simulink model "suspended_motion_test"  (R2014b)
settings: Solver=FixedStepDiscrete  StartTime=0.0  StopTime=inf  FixedStep=sample_time  RelTol=1e-3
undefined symbols (not defined in the file): A_angle_lat, A_lpf_accel, A_lpf_dtau, angle_midpoint_lat, B1_lpf_accel, B1_lpf_dtau, B2_lpf_accel, B2_lpf_dtau, back_left_triangle_period, back_left_triangle_wave_midpoint, back_left_triangle_wave_speed, back_right_triangle_period, back_right_triangle_wave_midpoint, back_right_triangle_wave_speed, boom_mount_angle, control_start_time, front_left_triangle_period, front_left_triangle_wave_midpoint, front_left_triangle_wave_speed, front_right_triangle_period, front_right_triangle_wave_midpoint, front_right_triangle_wave_speed, g, j_segments, k_ff, k_sea, kd_lateral, kd_motor, kd_sea_torque_flight, kd_sea_torque_stance, kp_lateral, kp_motor, kp_sea_torque_flight, kp_sea_torque_stance, lateral_offset, lateral_torque_ramp_time, m_leg_motor, max_sagittal_loaded_torque, max_sagittal_unloaded_torque, max_torque_lateral, maximum_lateral_angle, minimum_lateral_angle, sagittal_torque_ramp_time, sample_time, sea_control_torque_cmd_small_threshold, sea_offset_friction, sea_static_friction, stance_flight_torque_threshold, w_angle_lat
libraries: simulink x8
settings Model: xpc_rtwmakecfg_data=_xpcethercatlib_  BufferReuse=off  Creator=wmartin  LastModifiedBy=wmartin
settings SolverCC: EnableConcurrentExecution=on
settings DataIOCC: MaxDataPoints=1000000000  SaveFormat=StructureWithTime
settings OptimizationCC: BlockReduction=off  OptimizeBlockIOStorage=off  BufferReuse=off  GlobalBufferReuse=off  ExpressionFolding=off  ExpressionDepthLimit=2147483647  LocalBlockOutputs=off  SimCompilerOptimization=On
settings DebuggingCC: UnderspecifiedInitializationDetection=Classic  MergeDetectMultiDrivingBlocksExec=none  StateNameClashWarn=warning
settings HardwareCC: ProdIntDivRoundTo=Zero  ProdEndianess=LittleEndian  ProdLongLongMode=on  ProdHWDeviceType=Generic->32-bit x86 compatible
settings ModelReferenceCC: UpdateModelReferenceTargets=IfOutOfDate  EnableParallelModelReferenceBuilds=on
settings RTWCC: SystemTargetFile=slrt.tlc  TemplateMakefile=slrt_default_tmf  Description=Simulink Real-Time  RTWVerbose=off  ProcessScript=slrt_make_rtw_hook  RTWCompilerOptimization=On
settings CodeAppCC: MaxIdLength=256
settings SimulinkRealTimeCC: GeneratePreprocessorConditionals=Disable all  EnableShiftOperators=on  RL32LogBufSizeModifier=100000000

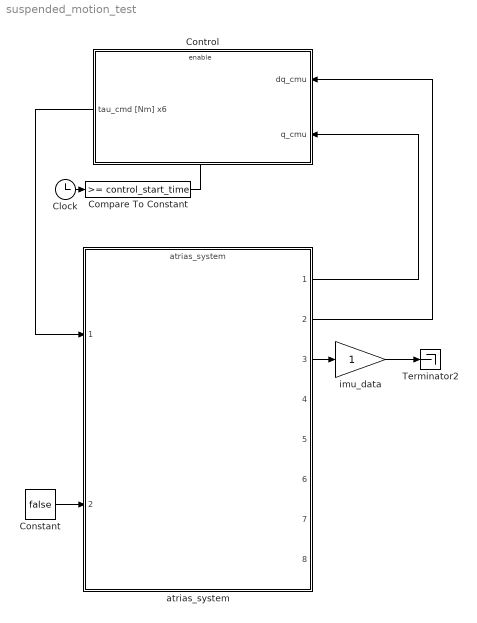
== system suspended_motion_test ==
  Clock : Clock
  Compare To Constant : simulink/Logic and Bit Operations/Compare To Constant  relop=>=  const=control_start_time  OutDataTypeStr=boolean
  Constant : Constant  Value=false
  Control : Subsystem
  Terminator2 : Terminator
  atrias_system : ModelReference  ModelNameDialog=atrias_system  SimulationMode=Normal  ModelReferenceVersion=1.2635  CopyOfModelName=atrias_system  DefaultDataLogging=on
  imu_data : Gain
  wires:
  Clock/1 -> Compare To Constant/1
  Compare To Constant/1 -> Control/Enable
  atrias_system/1 -> Control/2(q_cmu)
  atrias_system/2 -> Control/1(dq_cmu)
  Constant/1 -> atrias_system/2
  Control/1(tau_cmd [Nm] x6) -> atrias_system/1
  imu_data/1 -> Terminator2/1
  atrias_system/3 -> imu_data/1

== system suspended_motion_test/Control ==
  dq_cmu : Inport
  q_cmu : Inport  Port=2
  Enable : EnablePort  StatesWhenEnabling=reset
  Actuator Control : ModelReference  ModelNameDialog=actuator_control  SimulationMode=Normal  ModelReferenceVersion=1.25  CopyOfModelName=actuator_control  DefaultDataLogging=on
  Actuator Control old : Subsystem  Commented=on
  Behavior Control : Subsystem
  Constant : Constant  Value=[false false false false]  OutDataTypeStr=boolean
  tau_cmd [Nm] x6 : Outport  InitialOutput=[0 0 0 0 0 0]
  wires:
  q_cmu/1 -> Actuator Control/3, Behavior Control/2(q_cmu)
  dq_cmu/1 -> Actuator Control/4, Behavior Control/1(dq_cmu)
  Behavior Control/1(motor_torque_cmd) -> Actuator Control/1
  Actuator Control/1 -> tau_cmd [Nm] x6/1
  Constant/1 -> Actuator Control/2

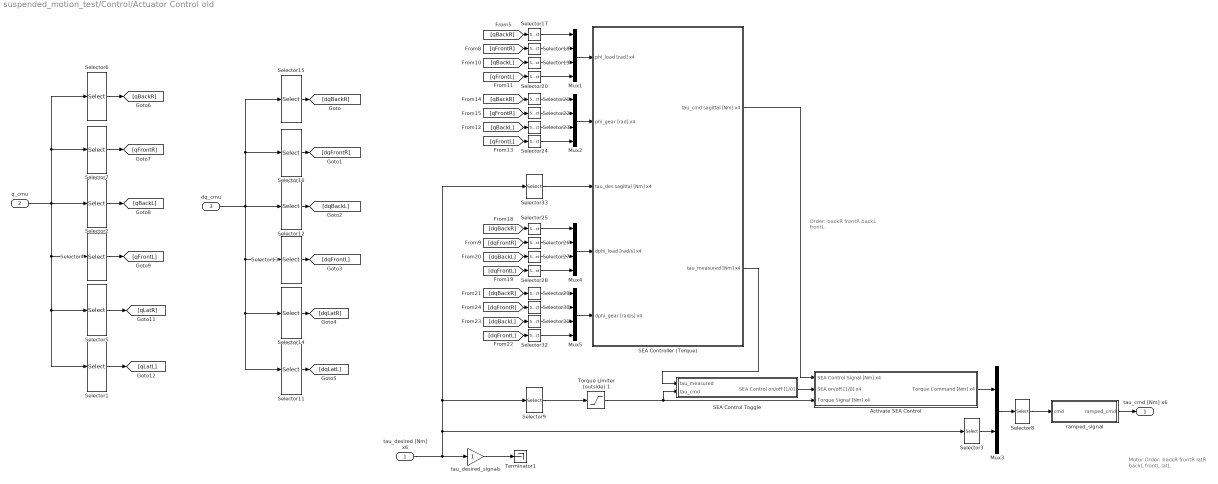
== system suspended_motion_test/Control/Actuator Control old ==
  note: Motor Order:
      |
      | backR
      | frontR
      | latR
      | backL
      | frontL
      | latL
  note: Order:
      | backR
      | frontR
      | backL
      | frontL
  tau_desired [Nm] x6 : Inport
  q_cmu : Inport  Port=2
  dq_cmu : Inport  Port=3
  Activate SEA Control : Subsystem
  Mux{1..2,4..5} (4 alike) : Mux
  Mux3 : Mux  Inputs=2
  SEA Control Toggle : Subsystem
  SEA Controller (Torque) : Subsystem
  Selector1 : Selector  InputPortWidth=13  Indices=[10]
  Selector11 : Selector  InputPortWidth=13  Indices=[10]
  Selector12 : Selector  InputPortWidth=13  Indices=[5 6]
  Selector13 : Selector  InputPortWidth=13  Indices=[7 8]
  Selector14 : Selector  InputPortWidth=13  Indices=[9]
  Selector15 : Selector  InputPortWidth=13  Indices=[1 2]
  Selector16 : Selector  InputPortWidth=13  Indices=[3 4]
  Selector{17..20,25..28} (8 alike) : Selector  InputPortWidth=2  Indices=[1]
  Selector2 : Selector  InputPortWidth=13  Indices=[5 6]
  Selector{21..24,29..32} (8 alike) : Selector  InputPortWidth=2  Indices=[2]
  Selector3 : Selector  InputPortWidth=6  Indices=[3 6]
  Selector33 : Selector  InputPortWidth=6  Indices=[1 2 4 5]
  Selector4 : Selector  InputPortWidth=13  Indices=[7 8]
  Selector5 : Selector  InputPortWidth=13  Indices=[9]
  Selector6 : Selector  InputPortWidth=13  Indices=[1 2]
  Selector7 : Selector  InputPortWidth=13  Indices=[3 4]
  Selector8 : Selector  InputPortWidth=6  Indices=[1 2 5 3 4 6]
  Selector9 : Selector  InputPortWidth=6  Indices=[1 2 4 5]
  Terminator1 : Terminator
  Torque Limiter (outside) 1 : Saturate  UpperLimit=max_sagittal_unloaded_torque  LowerLimit=-max_sagittal_unloaded_torque
      settings: AttributesFormatString=Hi: %<UpperLimit>\nLo: %<LowerLimit>
  ramped_signal : Subsystem
  tau_desired_signals : Gain  Description=xPCTag(1)=tau_cmd_signal;
  tau_cmd [Nm] x6 : Outport  InitialOutput=[0 0 0 0 0 0]
  wires:
  Mux3/1 -> Selector8/1
  Selector3/1 -> Mux3/2
  Selector33/1 -> SEA Controller (Torque)/3(tau_des sagittal [Nm] x4)
  [dqFrontL] -> Selector32/1
  [dqBackL] -> Selector31/1
  [dqFrontR] -> Selector30/1
  Selector32/1 -> Mux5/4
  Selector30/1 -> Mux5/2
  Selector31/1 -> Mux5/3
  Selector29/1 -> Mux5/1
  [dqBackR] -> Selector29/1
  Mux5/1 -> SEA Controller (Torque)/5(dphi_gear [rad/s] x4)
  [dqFrontL] -> Selector28/1
  [dqBackL] -> Selector27/1
  [dqFrontR] -> Selector26/1
  Selector28/1 -> Mux4/4
  Selector26/1 -> Mux4/2
  Selector27/1 -> Mux4/3
  Selector25/1 -> Mux4/1
  [dqBackR] -> Selector25/1
  Mux4/1 -> SEA Controller (Torque)/4(dphi_load [rad/s] x4)
  [qFrontL] -> Selector24/1
  [qBackL] -> Selector23/1
  [qFrontR] -> Selector22/1
  Selector24/1 -> Mux2/4
  Selector22/1 -> Mux2/2
  Selector23/1 -> Mux2/3
  Selector21/1 -> Mux2/1
  [qBackR] -> Selector21/1
  Mux2/1 -> SEA Controller (Torque)/2(phi_gear [rad] x4)
  [qFrontL] -> Selector20/1
  [qBackL] -> Selector19/1
  [qFrontR] -> Selector18/1
  Selector20/1 -> Mux1/4
  Selector18/1 -> Mux1/2
  Selector19/1 -> Mux1/3
  Selector17/1 -> Mux1/1
  [qBackR] -> Selector17/1
  Mux1/1 -> SEA Controller (Torque)/1(phi_load [rad] x4)
  Selector13/1 -> [dqFrontL]
  Selector12/1 -> [dqBackL]
  Selector16/1 -> [dqFrontR]
  Selector15/1 -> [dqBackR]
  Selector11/1 -> [dqLatL]
  Selector14/1 -> [dqLatR]
  dq_cmu/1 -> Selector11/1, Selector14/1, Selector13/1, Selector15/1, Selector16/1, Selector12/1
  Selector8/1 -> ramped_signal/1(cmd)
  q_cmu/1 -> Selector2/1, Selector7/1, Selector6/1, Selector4/1, Selector5/1, Selector1/1
  Selector4/1 -> [qFrontL]
  Selector2/1 -> [qBackL]
  Selector7/1 -> [qFrontR]
  Selector6/1 -> [qBackR]
  Selector1/1 -> [qLatL]
  Selector5/1 -> [qLatR]
  tau_desired_signals/1 -> Terminator1/1
  ramped_signal/1(ramped_cmd) -> tau_cmd [Nm] x6/1
  tau_desired [Nm] x6/1 -> Selector33/1, Selector9/1, Selector3/1, tau_desired_signals/1
  Activate SEA Control/1(Torque Command [Nm] x4) -> Mux3/1
  Torque Limiter (outside) 1/1 -> Activate SEA Control/3(Torque Signal [Nm] x4), SEA Control Toggle/2(tau_cmd)
  SEA Controller (Torque)/1(tau_cmd sagittal [Nm] x4) -> Activate SEA Control/1(SEA Control Signal [Nm] x4)
  SEA Control Toggle/1(SEA Control on/off [1/0]) -> Activate SEA Control/2("SEA on/off [1/0] x4 ")
  SEA Controller (Torque)/2(tau_measured [Nm] x4) -> SEA Control Toggle/1(tau_measured)
  Selector9/1 -> Torque Limiter (outside) 1/1

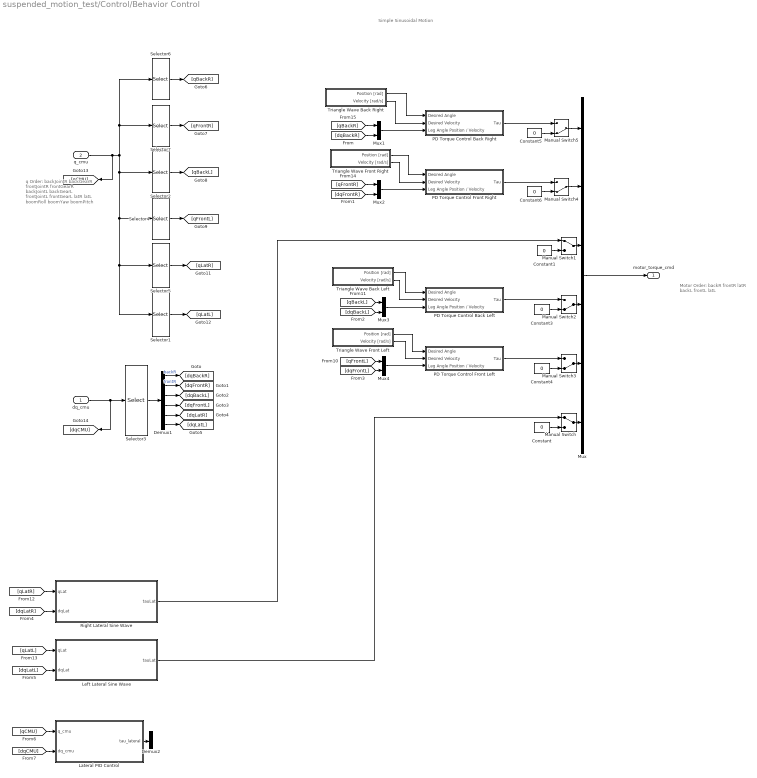
== system suspended_motion_test/Control/Behavior Control ==
  note: q Order:
      |
      | backJointR
      | backGearR
      | frontJointR
      | frontGearR
      |
      | backJointL
      | backGearL
      | frontJointL
      | frontGearL
      |
      | latR
      | latL
      |
      | boomRoll
      | boomYaw
      | boomPitch
  note: Motor Order:
      |
      | backR
      | frontR
      | latR
      | backL
      | frontL
      | latL
  note: Simple Sinusoidal Motion
  dq_cmu : Inport
  q_cmu : Inport  Port=2
  Constant{,1,3..6} (6 alike) : Constant  Value=0
  Demux1 : Demux  Outputs=6
  Demux2 : Demux  Outputs=2
  Lateral PID Control : Subsystem
  Left Lateral Sine Wave : Subsystem
  Manual Switch : ManualSwitch
  Manual Switch1 : ManualSwitch
  Manual Switch{2..5} (4 alike) : ManualSwitch  CurrentSetting=0
  Mux : Mux  Inputs=6
  Mux{1..4} (4 alike) : Mux  Inputs=2
  PD Torque Control Back Left : Subsystem
  PD Torque Control Back Right : Subsystem
  PD Torque Control Front Left : Subsystem
  PD Torque Control Front Right : Subsystem
  Right Lateral Sine Wave : Subsystem
  Selector1 : Selector  InputPortWidth=13  Indices=[10]
  Selector2 : Selector  InputPortWidth=13  Indices=[6]
  Selector3 : Selector  InputPortWidth=13  Indices=[2 4 6 8 9 10]
  Selector4 : Selector  InputPortWidth=13  Indices=[8]
  Selector5 : Selector  InputPortWidth=13  Indices=[9]
  Selector6 : Selector  InputPortWidth=13  Indices=[2]
  Selector7 : Selector  InputPortWidth=13  Indices=[4]
  Triangle Wave Back Left : Subsystem
  Triangle Wave Back Right : Subsystem
  Triangle Wave Front Left : Subsystem
  Triangle Wave Front Right : Subsystem
  motor_torque_cmd : Outport  OutputWhenDisabled=reset  InitialOutput=[0 0 0 0 0 0]
  wires:
  Mux/1 -> motor_torque_cmd/1
  dq_cmu/1 -> [dqCMU], Selector3/1
  Selector3/1 -> Demux1/1
  Left Lateral Sine Wave/1(tauLat) -> Manual Switch/1
  Manual Switch1/1 -> Mux/3
  Manual Switch/1 -> Mux/6
  Constant/1 -> Manual Switch/2
  Constant1/1 -> Manual Switch1/2
  Selector5/1 -> [qLatR]
  Selector1/1 -> [qLatL]
  Demux1/1 -> [dqBackR]  "backR"
  Demux1/2 -> [dqFrontR]  "frontR"
  Demux1/3 -> [dqBackL]
  Demux1/4 -> [dqFrontL]
  Demux1/5 -> [dqLatR]
  Demux1/6 -> [dqLatL]
  [dqLatL] -> Left Lateral Sine Wave/2(dqLat)
  Selector6/1 -> [qBackR]
  Selector7/1 -> [qFrontR]
  Selector2/1 -> [qBackL]
  Selector4/1 -> [qFrontL]
  q_cmu/1 -> [qCMU], Selector1/1, Selector5/1, Selector4/1, Selector2/1, Selector7/1, Selector6/1
  [qLatL] -> Left Lateral Sine Wave/1(qLat)
  PD Torque Control Back Right/1(Tau) -> Manual Switch5/1
  PD Torque Control Front Right/1(Tau) -> Manual Switch4/1
  Constant3/1 -> Manual Switch2/2
  Constant4/1 -> Manual Switch3/2
  Manual Switch3/1 -> Mux/5
  Manual Switch2/1 -> Mux/4
  [qBackR] -> Mux1/1
  [dqBackR] -> Mux1/2
  Mux1/1 -> PD Torque Control Back Right/3(Leg Angle Position / Velocity)
  [qFrontR] -> Mux2/1
  [dqFrontR] -> Mux2/2
  Mux2/1 -> PD Torque Control Front Right/3(Leg Angle Position / Velocity)
  [qBackL] -> Mux3/1
  [dqBackL] -> Mux3/2
  [qFrontL] -> Mux4/1
  [dqFrontL] -> Mux4/2
  Triangle Wave Front Right/1(Position [rad]) -> PD Torque Control Front Right/1(Desired Angle)
  Triangle Wave Front Right/2(Velocity [rad/s]) -> PD Torque Control Front Right/2(Desired Velocity)
  Triangle Wave Back Right/1(Position [rad]) -> PD Torque Control Back Right/1(Desired Angle)
  Triangle Wave Back Right/2(Velocity [rad/s]) -> PD Torque Control Back Right/2(Desired Velocity)
  PD Torque Control Back Left/1(Tau) -> Manual Switch2/1
  Triangle Wave Back Left/1(Position [rad]) -> PD Torque Control Back Left/1(Desired Angle)
  Triangle Wave Back Left/2(Velocity [rad/s]) -> PD Torque Control Back Left/2(Desired Velocity)
  Mux3/1 -> PD Torque Control Back Left/3(Leg Angle Position / Velocity)
  PD Torque Control Front Left/1(Tau) -> Manual Switch3/1
  Mux4/1 -> PD Torque Control Front Left/3(Leg Angle Position / Velocity)
  Triangle Wave Front Left/2(Velocity [rad/s]) -> PD Torque Control Front Left/2(Desired Velocity)
  Triangle Wave Front Left/1(Position [rad]) -> PD Torque Control Front Left/1(Desired Angle)
  Manual Switch4/1 -> Mux/2
  Manual Switch5/1 -> Mux/1
  Constant5/1 -> Manual Switch5/2
  Constant6/1 -> Manual Switch4/2
  [qLatR] -> Right Lateral Sine Wave/1(qLat)
  [dqLatR] -> Right Lateral Sine Wave/2(dqLat)
  Lateral PID Control/1(tau_lateral) -> Demux2/1
  [dqCMU] -> Lateral PID Control/2(dq_cmu)
  [qCMU] -> Lateral PID Control/1(q_cmu)
  Right Lateral Sine Wave/1(tauLat) -> Manual Switch1/1

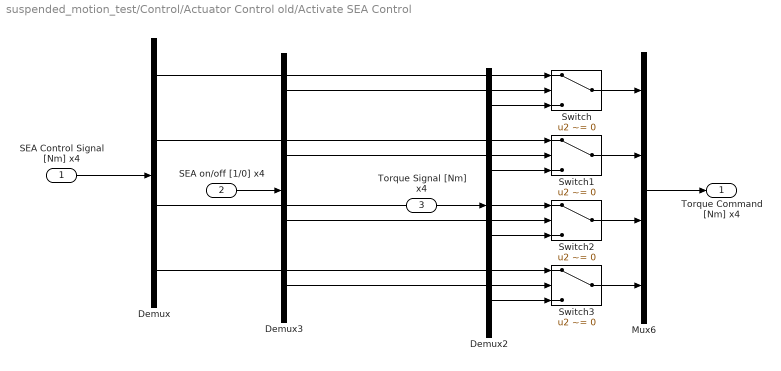
== system suspended_motion_test/Control/Actuator Control old/Activate SEA Control ==
  SEA Control Signal [Nm] x4 : Inport
  "SEA on/off [1/0] x4 " : Inport  Port=2
  Torque Signal [Nm] x4 : Inport  Port=3
  Demux : Demux
  Demux2 : Demux
  Demux3 : Demux
  Mux6 : Mux
  Switch{,1..3} (4 alike) : Switch  Criteria=u2 ~= 0
  Torque Command [Nm] x4 : Outport
  wires:
  Demux2/2 -> Switch1/3
  Demux2/1 -> Switch/3
  Demux/1 -> Switch/1
  Switch/1 -> Mux6/1
  Switch1/1 -> Mux6/2
  Switch3/1 -> Mux6/4
  Demux3/1 -> Switch/2
  Mux6/1 -> Torque Command [Nm] x4/1
  Demux3/3 -> Switch2/2
  Demux3/2 -> Switch1/2
  Demux/3 -> Switch2/1
  Switch2/1 -> Mux6/3
  Demux/4 -> Switch3/1
  Demux2/4 -> Switch3/3
  Demux3/4 -> Switch3/2
  Demux/2 -> Switch1/1
  Demux2/3 -> Switch2/3
  SEA Control Signal [Nm] x4/1 -> Demux/1
  "SEA on/off [1/0] x4 "/1 -> Demux3/1
  Torque Signal [Nm] x4/1 -> Demux2/1

== system suspended_motion_test/Control/Actuator Control old/SEA Control Toggle ==
  tau_measured : Inport
  tau_cmd : Inport  Port=2
  Abs : Abs
  Abs1 : Abs
  But Commanding a Small Torque? : simulink/Logic and Bit Operations/Compare To Constant  relop=<  const=sea_control_torque_cmd_small_threshold  OutDataTypeStr=boolean
  Logical Operator1 : Logic  AllPortsSameDT=off  OutDataTypeStr=boolean
  Logical Operator2 : Logic  Operator=NOT  AllPortsSameDT=off  OutDataTypeStr=boolean
  Measuring a Large Torque? (High Gains) : simulink/Logic and Bit Operations/Compare To Constant  relop=>=  const=stance_flight_torque_threshold  OutDataTypeStr=boolean
  SEA Control on/off [1/0] : Outport
  wires:
  Logical Operator2/1 -> SEA Control on/off [1/0]/1
  But Commanding a Small Torque?/1 -> Logical Operator1/2
  Logical Operator1/1 -> Logical Operator2/1
  tau_cmd/1 -> Abs/1
  Abs/1 -> But Commanding a Small Torque?/1
  tau_measured/1 -> Abs1/1
  Measuring a Large Torque? (High Gains)/1 -> Logical Operator1/1
  Abs1/1 -> Measuring a Large Torque? (High Gains)/1

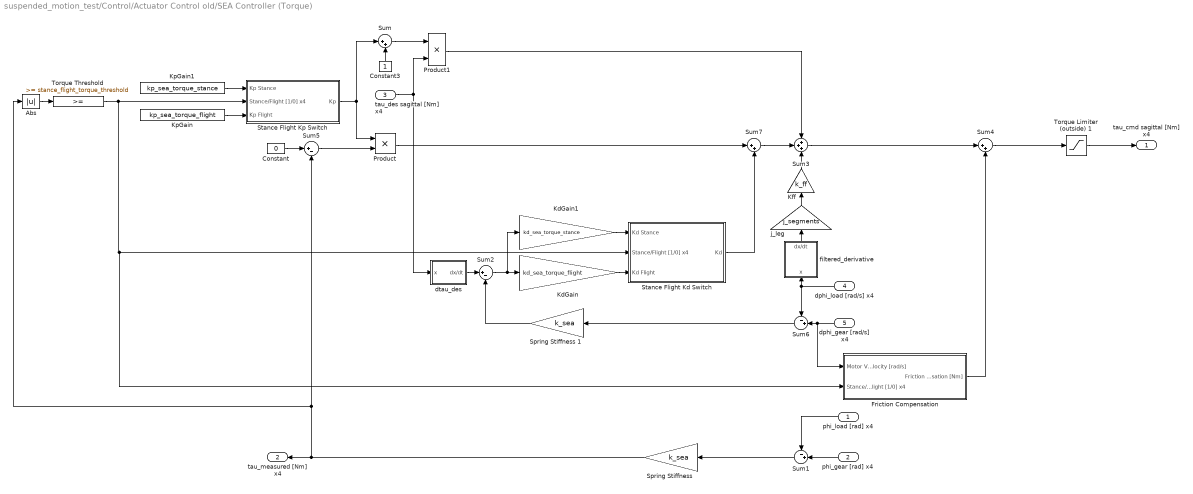
== system suspended_motion_test/Control/Actuator Control old/SEA Controller (Torque) ==
  phi_load [rad] x4 : Inport
  phi_gear [rad] x4 : Inport  Port=2
  tau_des sagittal [Nm] x4 : Inport  Port=3
  dphi_load [rad/s] x4 : Inport  Port=4
  dphi_gear [rad/s] x4 : Inport  Port=5
  Abs : Abs
  Constant : Constant  Value=0
  Constant3 : Constant
  Friction Compensation : Subsystem
  KdGain : Gain  Description=xPCTag(1)=kd_sea_torque;  Gain=kd_sea_torque_flight
  KdGain1 : Gain  Description=xPCTag(1)=kd_sea_torque;  Gain=kd_sea_torque_stance
  Kff : Gain  Gain=k_ff
  KpGain : Constant  Value=kp_sea_torque_flight  SampleTime=sample_time
  KpGain1 : Constant  Value=kp_sea_torque_stance  SampleTime=sample_time
  Product : Product  SampleTime=sample_time  RndMeth=Zero
  Product1 : Product  RndMeth=Zero
  Spring Stiffness : Gain  Gain=k_sea
  Spring Stiffness 1 : Gain  Gain=k_sea
  Stance Flight Kd Switch : Subsystem
  Stance Flight Kp Switch : Subsystem
  Sum : Sum  Inputs=|++  SampleTime=sample_time
  Sum1 : Sum  Inputs=-+|
  Sum2 : Sum  Inputs=|+-
  Sum3 : Sum  Inputs=+++
  Sum4 : Sum  Inputs=|++
  Sum5 : Sum  Inputs=|+-
  Sum6 : Sum  Inputs=-+|
  Sum7 : Sum  Inputs=|++
  Torque Limiter (outside) 1 : Saturate  UpperLimit=max_sagittal_loaded_torque  LowerLimit=-max_sagittal_loaded_torque
      settings: AttributesFormatString=Hi: %<UpperLimit>\nLo: %<LowerLimit>
  Torque Threshold : simulink/Logic and Bit Operations/Compare To Constant  relop=>=  const=stance_flight_torque_threshold  OutDataTypeStr=boolean
  dtau_des : Subsystem
  filtered_derivative : Subsystem
  j_leg : Gain  Description=xPCTag(1)=kd_sea_torque;  Gain=j_segments
  tau_cmd sagittal [Nm] x4 : Outport
  tau_measured [Nm] x4 : Outport  Port=2
  wires:
  Stance Flight Kd Switch/1(Kd) -> Sum7/2
  Sum4/1 -> Torque Limiter (outside) 1/1
  Friction Compensation/1(Friction Compensation [Nm]) -> Sum4/2
  Sum3/1 -> Sum4/1
  Abs/1 -> Torque Threshold/1
  Stance Flight Kp Switch/1(Kp) -> Product/1, Sum/1
  Spring Stiffness/1 -> tau_measured [Nm] x4/1, Abs/1, Sum5/2
  KdGain1/1 -> Stance Flight Kd Switch/1(Kd Stance)
  KpGain/1 -> Stance Flight Kp Switch/3(Kp Flight)
  Torque Threshold/1 -> Stance Flight Kp Switch/2(Stance/Flight [1/0] x4), Stance Flight Kd Switch/2(Stance/Flight [1/0] x4), Friction Compensation/2(Stance/Flight [1/0] x4)
  KpGain1/1 -> Stance Flight Kp Switch/1(Kp Stance)
  Sum1/1 -> Spring Stiffness/1
  tau_des sagittal [Nm] x4/1 -> dtau_des/1(x), Product1/2
  Product1/1 -> Sum3/1
  phi_load [rad] x4/1 -> Sum1/1
  phi_gear [rad] x4/1 -> Sum1/2
  Constant/1 -> Sum5/1
  dtau_des/1(dx/dt) -> Sum2/1
  Sum6/1 -> Spring Stiffness 1/1
  Spring Stiffness 1/1 -> Sum2/2
  dphi_load [rad/s] x4/1 -> Sum6/1, filtered_derivative/1(x)
  dphi_gear [rad/s] x4/1 -> Sum6/2, Friction Compensation/1(Motor Velocity [rad/s])
  Sum2/1 -> KdGain/1, KdGain1/1
  Sum5/1 -> Product/2
  Product/1 -> Sum7/1
  KdGain/1 -> Stance Flight Kd Switch/3(Kd Flight)
  Sum7/1 -> Sum3/2
  Constant3/1 -> Sum/2
  Sum/1 -> Product1/1
  filtered_derivative/1(dx/dt) -> j_leg/1
  j_leg/1 -> Kff/1
  Torque Limiter (outside) 1/1 -> tau_cmd sagittal [Nm] x4/1
  Kff/1 -> Sum3/3

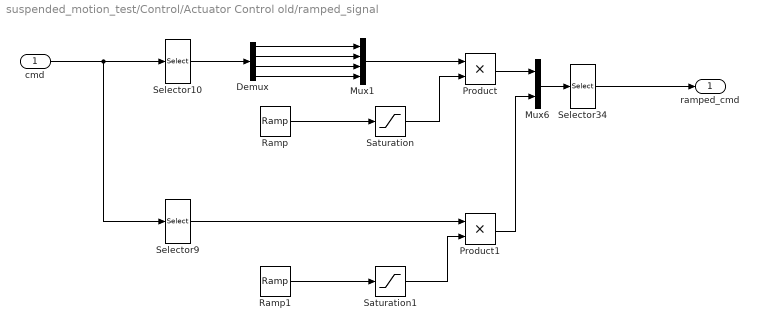
== system suspended_motion_test/Control/Actuator Control old/ramped_signal ==
  cmd : Inport
  Demux : Demux
  Mux1 : Mux
  Mux6 : Mux  Inputs=2
  Product : Product  RndMeth=Zero
  Product1 : Product  RndMeth=Zero
  Ramp : simulink/Sources/Ramp  slope=1/sagittal_torque_ramp_time  start=sagittal_starting_time  X0=0
      settings: AttributesFormatString=Start: %<start>\nSlope: %<slope>
  Ramp1 : simulink/Sources/Ramp  slope=1/lateral_torque_ramp_time  start=control_start_time  X0=0
      settings: AttributesFormatString=Start: %<start>\nSlope: %<slope>
  Saturation : Saturate  UpperLimit=1  LowerLimit=0
      settings: AttributesFormatString=Hi: %<UpperLimit>\nLo: %<LowerLimit>
  Saturation1 : Saturate  UpperLimit=1  LowerLimit=0
      settings: AttributesFormatString=Hi: %<UpperLimit>\nLo: %<LowerLimit>
  Selector10 : Selector  InputPortWidth=6  Indices=[1 2 4 5]
  Selector34 : Selector  InputPortWidth=6  Indices=[1 2 5 3 4 6]
  Selector9 : Selector  InputPortWidth=6  Indices=[3 6]
  ramped_cmd : Outport
  wires:
  Selector9/1 -> Product1/1
  Saturation1/1 -> Product1/2
  Ramp1/1 -> Saturation1/1
  Saturation/1 -> Product/2
  Ramp/1 -> Saturation/1
  Product/1 -> Mux6/1
  cmd/1 -> Selector10/1, Selector9/1
  Product1/1 -> Mux6/2
  Selector34/1 -> ramped_cmd/1
  Selector10/1 -> Demux/1
  Mux6/1 -> Selector34/1
  Demux/1 -> Mux1/1
  Demux/2 -> Mux1/2
  Mux1/1 -> Product/1
  Demux/4 -> Mux1/4
  Demux/3 -> Mux1/3

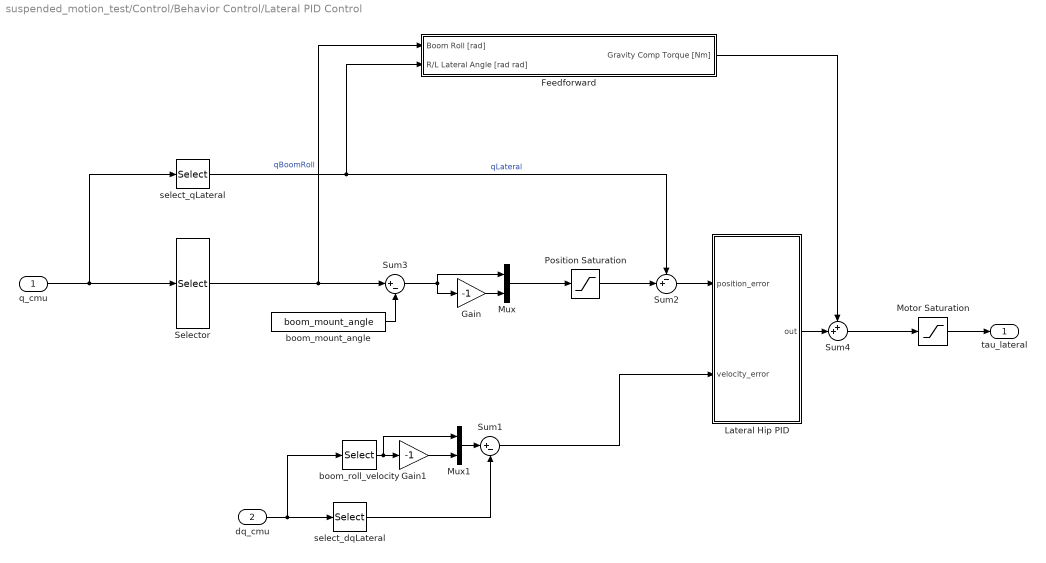
== system suspended_motion_test/Control/Behavior Control/Lateral PID Control ==
  q_cmu : Inport
  dq_cmu : Inport  Port=2
  Feedforward : Subsystem
  Gain : Gain  Gain=-1
  Gain1 : Gain  Gain=-1
  Lateral Hip PID : Subsystem
  Motor Saturation : Saturate  UpperLimit=max_torque_lateral  LowerLimit=-max_torque_lateral
      settings: AttributesFormatString=Top: %<UpperLimit>\nBottom: %<LowerLimit>
  Mux : Mux  Inputs=2
  Mux1 : Mux  Inputs=2
  Position Saturation : Saturate  UpperLimit=maximum_lateral_angle  LowerLimit=minimum_lateral_angle
      settings: AttributesFormatString=Top: %<UpperLimit>\nBottom: %<LowerLimit>
  Selector : Selector  InputPortWidth=13  Indices=[11]
  Sum1 : Sum  Inputs=|+-
  Sum2 : Sum  Inputs=-+|
  Sum3 : Sum  Inputs=|+-
  Sum4 : Sum  Inputs=++|
  boom_mount_angle : Constant  Value=boom_mount_angle
  boom_roll_velocity : Selector  InputPortWidth=13  Indices=[11]
  select_dqLateral : Selector  InputPortWidth=13  Indices=[9 10]
  select_qLateral : Selector  InputPortWidth=13  Indices=[9 10]
  tau_lateral : Outport
  wires:
  Lateral Hip PID/1(out) -> Sum4/2
  Position Saturation/1 -> Sum2/2
  Sum4/1 -> Motor Saturation/1
  Sum2/1 -> Lateral Hip PID/1(position_error)
  select_dqLateral/1 -> Sum1/2
  dq_cmu/1 -> select_dqLateral/1, boom_roll_velocity/1
  boom_roll_velocity/1 -> Mux1/1, Gain1/1
  Sum1/1 -> Lateral Hip PID/2(velocity_error)
  Gain/1 -> Mux/2
  Mux/1 -> Position Saturation/1
  select_qLateral/1 -> Feedforward/2(R/L Lateral Angle [rad rad]), Sum2/1  "qLateral"
  Motor Saturation/1 -> tau_lateral/1
  Sum3/1 -> Mux/1, Gain/1
  Mux1/1 -> Sum1/1
  Gain1/1 -> Mux1/2
  Feedforward/1(Gravity Comp Torque [Nm]) -> Sum4/1
  boom_mount_angle/1 -> Sum3/2
  q_cmu/1 -> select_qLateral/1, Selector/1
  Selector/1 -> Feedforward/1(Boom Roll [rad]), Sum3/1  "qBoomRoll"

== system suspended_motion_test/Control/Behavior Control/Left Lateral Sine Wave ==
  qLat : Inport
  dqLat : Inport  Port=2
  Hip Roll PD : Subsystem
  Left Theta Desired : Sin  Amplitude=A_angle_lat  Bias=angle_midpoint_lat  Frequency=w_angle_lat  SampleTime=0
  Mux1 : Mux  Inputs=2
  Mux2 : Mux  Inputs=2
  dTheta Desired : Sin  Amplitude=A_angle_lat*w_angle_lat  Frequency=w_angle_lat  Phase=pi/2  SampleTime=0
  qLatSignal : Gain
  tauLat : Outport
  wires:
  dqLat/1 -> Mux2/2
  Mux2/1 -> Hip Roll PD/2(Position / Velocity)
  Hip Roll PD/1(tauLat) -> tauLat/1
  qLat/1 -> qLatSignal/1
  qLatSignal/1 -> Mux2/1
  Mux1/1 -> Hip Roll PD/1(Desired Position / Velocity)
  Left Theta Desired/1 -> Mux1/1
  dTheta Desired/1 -> Mux1/2

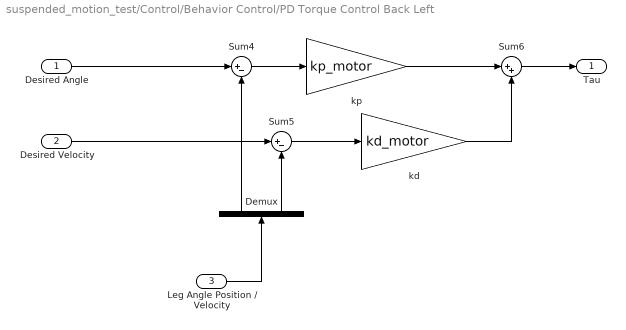
== system suspended_motion_test/Control/Behavior Control/PD Torque Control Back Left ==
  Desired Angle : Inport
  Desired Velocity : Inport  Port=2
  Leg Angle Position / Velocity : Inport  Port=3
  Demux : Demux  Outputs=2
  Sum4 : Sum  Inputs=|+-
  Sum5 : Sum  Inputs=|+-
  Sum6 : Sum  Inputs=|++
  kd : Gain  Gain=kd_motor
  kp : Gain  Gain=kp_motor
  Tau : Outport
  wires:
  kd/1 -> Sum6/2
  Demux/2 -> Sum5/2
  kp/1 -> Sum6/1
  Sum5/1 -> kd/1
  Sum4/1 -> kp/1
  Desired Velocity/1 -> Sum5/1
  Leg Angle Position / Velocity/1 -> Demux/1
  Demux/1 -> Sum4/2
  Desired Angle/1 -> Sum4/1
  Sum6/1 -> Tau/1

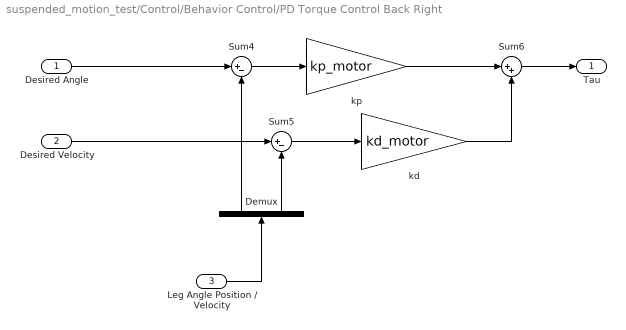
== system suspended_motion_test/Control/Behavior Control/PD Torque Control Back Right ==
  Desired Angle : Inport
  Desired Velocity : Inport  Port=2
  Leg Angle Position / Velocity : Inport  Port=3
  Demux : Demux  Outputs=2
  Sum4 : Sum  Inputs=|+-
  Sum5 : Sum  Inputs=|+-
  Sum6 : Sum  Inputs=|++
  kd : Gain  Gain=kd_motor
  kp : Gain  Gain=kp_motor
  Tau : Outport
  wires:
  Sum6/1 -> Tau/1
  Desired Angle/1 -> Sum4/1
  Demux/1 -> Sum4/2
  Leg Angle Position / Velocity/1 -> Demux/1
  Desired Velocity/1 -> Sum5/1
  Sum4/1 -> kp/1
  Sum5/1 -> kd/1
  kp/1 -> Sum6/1
  Demux/2 -> Sum5/2
  kd/1 -> Sum6/2

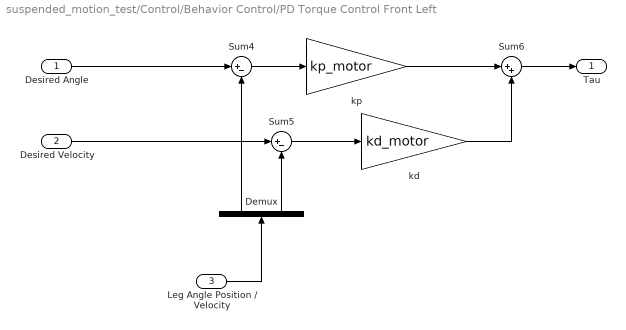
== system suspended_motion_test/Control/Behavior Control/PD Torque Control Front Left ==
  Desired Angle : Inport
  Desired Velocity : Inport  Port=2
  Leg Angle Position / Velocity : Inport  Port=3
  Demux : Demux  Outputs=2
  Sum4 : Sum  Inputs=|+-
  Sum5 : Sum  Inputs=|+-
  Sum6 : Sum  Inputs=|++
  kd : Gain  Gain=kd_motor
  kp : Gain  Gain=kp_motor
  Tau : Outport
  wires:
  Sum6/1 -> Tau/1
  Desired Angle/1 -> Sum4/1
  Demux/1 -> Sum4/2
  Leg Angle Position / Velocity/1 -> Demux/1
  Desired Velocity/1 -> Sum5/1
  Sum4/1 -> kp/1
  Sum5/1 -> kd/1
  kp/1 -> Sum6/1
  Demux/2 -> Sum5/2
  kd/1 -> Sum6/2

== system suspended_motion_test/Control/Behavior Control/PD Torque Control Front Right ==
  Desired Angle : Inport
  Desired Velocity : Inport  Port=2
  Leg Angle Position / Velocity : Inport  Port=3
  Demux : Demux  Outputs=2
  Sum4 : Sum  Inputs=|+-
  Sum5 : Sum  Inputs=|+-
  Sum6 : Sum  Inputs=|++
  kd : Gain  Gain=kd_motor
  kp : Gain  Gain=kp_motor
  Tau : Outport
  wires:
  kd/1 -> Sum6/2
  Demux/2 -> Sum5/2
  kp/1 -> Sum6/1
  Sum5/1 -> kd/1
  Sum4/1 -> kp/1
  Desired Velocity/1 -> Sum5/1
  Leg Angle Position / Velocity/1 -> Demux/1
  Demux/1 -> Sum4/2
  Desired Angle/1 -> Sum4/1
  Sum6/1 -> Tau/1

== system suspended_motion_test/Control/Behavior Control/Right Lateral Sine Wave ==
  qLat : Inport
  dqLat : Inport  Port=2
  Hip Roll PD : Subsystem
  Left Theta Desired : Sin  Amplitude=A_angle_lat  Bias=angle_midpoint_lat  Frequency=w_angle_lat  SampleTime=0
  Mux1 : Mux  Inputs=2
  Mux2 : Mux  Inputs=2
  dTheta Desired : Sin  Amplitude=A_angle_lat*w_angle_lat  Frequency=w_angle_lat  Phase=pi/2  SampleTime=0
  qLatSignal : Gain
  tauLat : Outport
  wires:
  dTheta Desired/1 -> Mux1/2
  Left Theta Desired/1 -> Mux1/1
  Mux1/1 -> Hip Roll PD/1(Desired Position / Velocity)
  qLatSignal/1 -> Mux2/1
  qLat/1 -> qLatSignal/1
  Hip Roll PD/1(tauLat) -> tauLat/1
  Mux2/1 -> Hip Roll PD/2(Position / Velocity)
  dqLat/1 -> Mux2/2

== system suspended_motion_test/Control/Behavior Control/Triangle Wave Back Left ==
  Constant1 : Constant  Value=0
  Constant5 : Constant  Value=-1
  Constant6 : Constant
  Direction : DiscretePulseGenerator  PulseType=Time based  Period=back_left_triangle_period  PulseWidth=50  PhaseDelay=back_left_triangle_period/4
  Manual Switch : ManualSwitch
  Speed : Gain  Gain=back_left_triangle_wave_speed
  Switch : Switch  Criteria=u2 ~= 0
  Triangle Wave : DiscreteIntegrator  InitialCondition=back_left_triangle_wave_midpoint  InitialConditionSetting=State (most efficient)  SampleTime=sample_time
  Position [rad] : Outport
  Velocity [rad/s] : Outport  Port=2
  wires:
  Triangle Wave/1 -> Position [rad]/1
  Constant5/1 -> Switch/3
  Manual Switch/1 -> Velocity [rad/s]/1, Triangle Wave/1
  Direction/1 -> Switch/2
  Switch/1 -> Speed/1
  Constant6/1 -> Switch/1
  Constant1/1 -> Manual Switch/2
  Speed/1 -> Manual Switch/1

== system suspended_motion_test/Control/Behavior Control/Triangle Wave Back Right ==
  Constant1 : Constant  Value=0
  Constant5 : Constant  Value=-1
  Constant6 : Constant
  Direction : DiscretePulseGenerator  PulseType=Time based  Period=back_right_triangle_period  PulseWidth=50  PhaseDelay=back_right_triangle_period/4
  Manual Switch : ManualSwitch
  Speed : Gain  Gain=back_right_triangle_wave_speed
  Switch : Switch  Criteria=u2 ~= 0
  Triangle Wave : DiscreteIntegrator  InitialCondition=back_right_triangle_wave_midpoint  InitialConditionSetting=State (most efficient)  SampleTime=sample_time
  Position [rad] : Outport
  Velocity [rad/s] : Outport  Port=2
  wires:
  Constant6/1 -> Switch/1
  Switch/1 -> Speed/1
  Direction/1 -> Switch/2
  Manual Switch/1 -> Velocity [rad/s]/1, Triangle Wave/1
  Constant5/1 -> Switch/3
  Triangle Wave/1 -> Position [rad]/1
  Speed/1 -> Manual Switch/1
  Constant1/1 -> Manual Switch/2

== system suspended_motion_test/Control/Behavior Control/Triangle Wave Front Left ==
  Constant1 : Constant  Value=0
  Constant5 : Constant  Value=-1
  Constant6 : Constant
  Direction : DiscretePulseGenerator  PulseType=Time based  Period=front_left_triangle_period  PulseWidth=50  PhaseDelay=front_left_triangle_period/4
  Manual Switch : ManualSwitch
  Speed : Gain  Gain=front_left_triangle_wave_speed
  Switch : Switch  Criteria=u2 ~= 0
  Triangle Wave : DiscreteIntegrator  InitialCondition=front_left_triangle_wave_midpoint  InitialConditionSetting=State (most efficient)  SampleTime=sample_time
  Position [rad] : Outport
  Velocity [rad/s] : Outport  Port=2
  wires:
  Constant6/1 -> Switch/1
  Switch/1 -> Speed/1
  Direction/1 -> Switch/2
  Manual Switch/1 -> Velocity [rad/s]/1, Triangle Wave/1
  Constant5/1 -> Switch/3
  Triangle Wave/1 -> Position [rad]/1
  Constant1/1 -> Manual Switch/2
  Speed/1 -> Manual Switch/1

== system suspended_motion_test/Control/Behavior Control/Triangle Wave Front Right ==
  Constant1 : Constant  Value=0
  Constant5 : Constant  Value=-1
  Constant6 : Constant
  Direction : DiscretePulseGenerator  PulseType=Time based  Period=front_right_triangle_period  PulseWidth=50  PhaseDelay=front_right_triangle_period/4
  Manual Switch : ManualSwitch
  Speed : Gain  Gain=front_right_triangle_wave_speed
  Switch : Switch  Criteria=u2 ~= 0
  Triangle Wave : DiscreteIntegrator  InitialCondition=front_right_triangle_wave_midpoint  InitialConditionSetting=State (most efficient)  SampleTime=sample_time
  Position [rad] : Outport
  Velocity [rad/s] : Outport  Port=2
  wires:
  Triangle Wave/1 -> Position [rad]/1
  Constant5/1 -> Switch/3
  Manual Switch/1 -> Velocity [rad/s]/1, Triangle Wave/1
  Direction/1 -> Switch/2
  Switch/1 -> Speed/1
  Constant6/1 -> Switch/1
  Constant1/1 -> Manual Switch/2
  Speed/1 -> Manual Switch/1

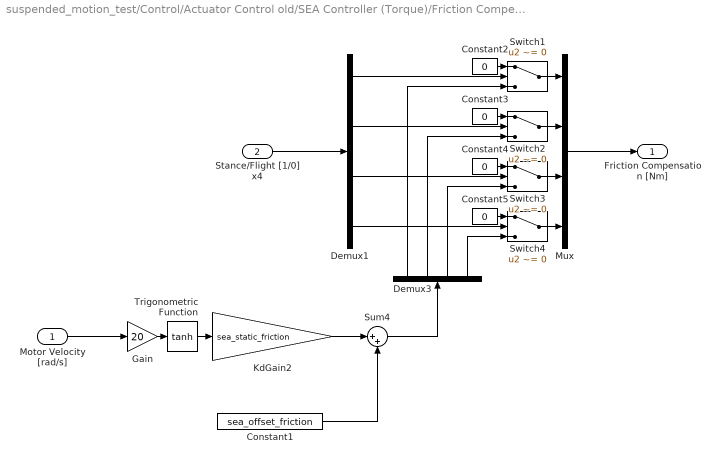
== system suspended_motion_test/Control/Actuator Control old/SEA Controller (Torque)/Friction Compensation ==
  Motor Velocity [rad/s] : Inport
  Stance/Flight [1/0] x4 : Inport  Port=2
  Constant1 : Constant  Value=sea_offset_friction
  Constant{2..5} (4 alike) : Constant  Value=0
  Demux1 : Demux
  Demux3 : Demux
  Gain : Gain  Gain=20
  KdGain2 : Gain  Description=xPCTag(1)=kd_sea_torque;  Gain=sea_static_friction
  Mux : Mux
  Sum4 : Sum  Inputs=|++
  Switch{1..4} (4 alike) : Switch  Criteria=u2 ~= 0
  Trigonometric Function : Trigonometry  Operator=tanh
  Friction Compensation [Nm] : Outport
  wires:
  Mux/1 -> Friction Compensation [Nm]/1
  Sum4/1 -> Demux3/1
  Constant5/1 -> Switch4/1
  Constant4/1 -> Switch3/1
  Constant3/1 -> Switch2/1
  Constant2/1 -> Switch1/1
  Stance/Flight [1/0] x4/1 -> Demux1/1
  Demux3/1 -> Switch1/3
  Demux3/2 -> Switch2/3
  Demux3/3 -> Switch3/3
  Demux3/4 -> Switch4/3
  Demux1/1 -> Switch1/2
  Switch1/1 -> Mux/1
  Switch4/1 -> Mux/4
  Switch3/1 -> Mux/3
  Switch2/1 -> Mux/2
  Demux1/2 -> Switch2/2
  Demux1/3 -> Switch3/2
  Demux1/4 -> Switch4/2
  Motor Velocity [rad/s]/1 -> Gain/1
  Gain/1 -> Trigonometric Function/1
  Trigonometric Function/1 -> KdGain2/1
  KdGain2/1 -> Sum4/1
  Constant1/1 -> Sum4/2

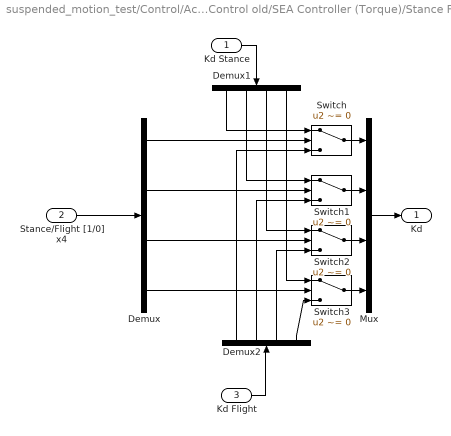
== system suspended_motion_test/Control/Actuator Control old/SEA Controller (Torque)/Stance Flight Kd Switch ==
  Kd Stance : Inport
  Stance/Flight [1/0] x4 : Inport  Port=2
  Kd Flight : Inport  Port=3
  Demux : Demux
  Demux1 : Demux
  Demux2 : Demux
  Mux : Mux
  Switch{,1..3} (4 alike) : Switch  Criteria=u2 ~= 0
  Kd : Outport
  wires:
  Demux2/1 -> Switch/3
  Demux2/2 -> Switch1/3
  Demux2/3 -> Switch2/3
  Demux2/4 -> Switch3/3
  Kd Flight/1 -> Demux2/1
  Demux1/4 -> Switch3/1
  Demux1/3 -> Switch2/1
  Demux1/2 -> Switch1/1
  Demux1/1 -> Switch/1
  Kd Stance/1 -> Demux1/1
  Demux/1 -> Switch/2
  Switch/1 -> Mux/1
  Mux/1 -> Kd/1
  Stance/Flight [1/0] x4/1 -> Demux/1
  Switch3/1 -> Mux/4
  Switch2/1 -> Mux/3
  Switch1/1 -> Mux/2
  Demux/2 -> Switch1/2
  Demux/3 -> Switch2/2
  Demux/4 -> Switch3/2

== system suspended_motion_test/Control/Actuator Control old/SEA Controller (Torque)/Stance Flight Kp Switch ==
  Kp Stance : Inport
  Stance/Flight [1/0] x4 : Inport  Port=2
  Kp Flight : Inport  Port=3
  Demux : Demux
  Mux : Mux
  Switch{,1..3} (4 alike) : Switch  Criteria=u2 ~= 0
  Kp : Outport
  wires:
  Demux/4 -> Switch3/2
  Demux/3 -> Switch2/2
  Demux/2 -> Switch1/2
  Switch1/1 -> Mux/2
  Switch2/1 -> Mux/3
  Switch3/1 -> Mux/4
  Stance/Flight [1/0] x4/1 -> Demux/1
  Mux/1 -> Kp/1
  Switch/1 -> Mux/1
  Demux/1 -> Switch/2
  Kp Stance/1 -> Switch/1, Switch1/1, Switch2/1, Switch3/1
  Kp Flight/1 -> Switch1/3, Switch2/3, Switch3/3, Switch/3

== system suspended_motion_test/Control/Actuator Control old/SEA Controller (Torque)/dtau_des ==
  x : Inport
  Gain1 : Gain  Gain=1/sample_time
  difference : simulink/Discrete/Difference  ICPrevInput=0.0  InputProcessing=Inherited  OutMin=[]  OutMax=[]  OutDataType=fixdt(1, 16)  OutScaling=2^-10  DoSatur=off
  two_pole_filter : DiscreteTransferFcn  Numerator=[A_lpf_dtau 0 0]  Denominator=[1 B1_lpf_dtau B2_lpf_dtau]  SampleTime=sample_time
  dx/dt : Outport
  wires:
  Gain1/1 -> difference/1
  difference/1 -> two_pole_filter/1
  x/1 -> Gain1/1
  two_pole_filter/1 -> dx/dt/1

== system suspended_motion_test/Control/Actuator Control old/SEA Controller (Torque)/filtered_derivative ==
  x : Inport
  Gain1 : Gain  Gain=1/sample_time
  difference : simulink/Discrete/Difference  ICPrevInput=0.0  InputProcessing=Inherited  OutMin=[]  OutMax=[]  OutDataType=fixdt(1, 16)  OutScaling=2^-10  DoSatur=off
  two_pole_filter : DiscreteTransferFcn  Numerator=[A_lpf_accel 0 0]  Denominator=[1 B1_lpf_accel B2_lpf_accel]  SampleTime=sample_time
  dx/dt : Outport
  wires:
  two_pole_filter/1 -> dx/dt/1
  x/1 -> Gain1/1
  difference/1 -> two_pole_filter/1
  Gain1/1 -> difference/1

== system suspended_motion_test/Control/Behavior Control/Lateral PID Control/Feedforward ==
  Boom Roll [rad] : Inport
  R/L Lateral Angle [rad rad] : Inport  Port=2
  -mgd : Gain  Gain=m_leg_motor*g*lateral_offset
  Gain2 : Gain  Gain=[-1 1]
  Sum1 : Sum  Inputs=++|
  Sum3 : Sum  Inputs=++|
  boom_mount_angle : Constant  Value=boom_mount_angle
  sin : Trigonometry  Operator=cos
  Gravity Comp Torque [Nm] : Outport
  wires:
  boom_mount_angle/1 -> Sum1/1
  -mgd/1 -> Gravity Comp Torque [Nm]/1
  sin/1 -> -mgd/1
  R/L Lateral Angle [rad rad]/1 -> Sum3/2
  Boom Roll [rad]/1 -> Sum1/2
  Sum1/1 -> Gain2/1
  Gain2/1 -> Sum3/1
  Sum3/1 -> sin/1

== system suspended_motion_test/Control/Behavior Control/Lateral PID Control/Lateral Hip PID ==
  position_error : Inport
  velocity_error : Inport  Port=2
  Sum : Sum  Inputs=++|
  kd_lateral : Gain  Description=xPCTag(1)=kd_lateral;  Gain=kd_lateral
  kp_lateral : Gain  Description=xPCTag(1)=kp_lateral;  Gain=kp_lateral
  out : Outport
  wires:
  velocity_error/1 -> kd_lateral/1
  kp_lateral/1 -> Sum/2
  position_error/1 -> kp_lateral/1
  Sum/1 -> out/1
  kd_lateral/1 -> Sum/1

== system suspended_motion_test/Control/Behavior Control/Left Lateral Sine Wave/Hip Roll PD ==
  Desired Position / Velocity : Inport
  Position / Velocity : Inport  Port=2
  Demux : Demux  Outputs=2
  Demux1 : Demux  Outputs=2
  Gain4 : Gain  Gain=kp_lateral
  Gain5 : Gain  Gain=kd_lateral
  Sum1 : Sum  Inputs=|+-
  Sum4 : Sum  Inputs=|+-
  Sum6 : Sum  Inputs=|++
  tauLat : Outport
  wires:
  Sum6/1 -> tauLat/1
  Demux/1 -> Sum4/2  "position"
  Position / Velocity/1 -> Demux/1
  Sum4/1 -> Gain4/1
  Sum1/1 -> Gain5/1
  Gain4/1 -> Sum6/1
  Demux/2 -> Sum1/2  "velocity"
  Gain5/1 -> Sum6/2
  Demux1/2 -> Sum1/1
  Desired Position / Velocity/1 -> Demux1/1
  Demux1/1 -> Sum4/1

== system suspended_motion_test/Control/Behavior Control/Right Lateral Sine Wave/Hip Roll PD ==
  Desired Position / Velocity : Inport
  Position / Velocity : Inport  Port=2
  Demux : Demux  Outputs=2
  Demux1 : Demux  Outputs=2
  Gain4 : Gain  Gain=kp_lateral
  Gain5 : Gain  Gain=kd_lateral
  Sum1 : Sum  Inputs=|+-
  Sum4 : Sum  Inputs=|+-
  Sum6 : Sum  Inputs=|++
  tauLat : Outport
  wires:
  Demux1/1 -> Sum4/1
  Desired Position / Velocity/1 -> Demux1/1
  Demux1/2 -> Sum1/1
  Gain5/1 -> Sum6/2
  Demux/2 -> Sum1/2  "velocity"
  Gain4/1 -> Sum6/1
  Sum1/1 -> Gain5/1
  Sum4/1 -> Gain4/1
  Position / Velocity/1 -> Demux/1
  Demux/1 -> Sum4/2  "position"
  Sum6/1 -> tauLat/1
